simulink library "tqd"  (R2021b)
settings: Solver=VariableStepAuto  StartTime=0.0  StopTime=10.0  RelTol=1e-3
undefined symbols (not defined in the file or in its folder): ATQD_APSDecReq_X_kph, ATQD_APSDecReq_Y_mps2, ATQD_APSDecReqCMD_X_kph, ATQD_APSDecReqTs_X_pct, ATQD_APSDecTimeGain_X_Deg, ATQD_APSDecTimeGain_Y_s, ATQD_APSReqLowSpd_X_Deg, ATQD_AutoHoldReleaseBPS_X_Deg, ATQD_AWDLoadTrqnsGain_X_kg, ATQD_AWDLoadTrqnsGain_Y_pct, ATQD_BOSEnBPSPosn_X_kph, ATQD_BOSMap_X_rpm, ATQD_BOSMap_Y_pct, ATQD_CreepBaseTqD_X_kph, ATQD_CreepBaseTqD_Y_Deg, ATQD_CreepBaseTqR_X_kph, ATQD_CreepBaseTqR_Y_Deg, ATQD_CreepBPSDisPosn_X_Deg, ATQD_CreepBPSDisPosnR_X_Deg, ATQD_CreepBPSEnPosn_X_Deg, ATQD_CreepBPSEnPosnR_X_Deg, ATQD_CreepDeltaTq_X_kph, ATQD_CreepIterm_X_kph, ATQD_CreepIterm_Y_kph, ATQD_CreepItermMaxLimit_X_pct, ATQD_CreepPreloadTime_X_kph, ATQD_CreepPreloadTq_X_kph, ATQD_CreepPreloadTq_Y_s, ATQD_CreepProtTq_X_Deg, ATQD_CreepPterm_X_kph, ATQD_ECOTqMapD_X_rpm, ATQD_ECOTqMapD_Y_pct, ATQD_EOPDTqMapDCon_X_rpm, ATQD_EOPDTqMapDCon_Y_Deg, ATQD_EstInitVehWeight_X_c, ATQD_LHMRollGenMapD_X_rpm, ATQD_LHMRollGenMapD_Y_rpm, ATQD_LHMTqMapD_X_rpm, ATQD_LHMTqMapD_Y_pct, ATQD_NL1TqMapD_X_rpm, ATQD_NL1TqMapD_Y_pct, ATQD_NOPDTqMapDCon_X_rpm, ATQD_NOPDTqMapDCon_Y_Deg, ATQD_NRMRrEDUSpRat_X_rpm, ATQD_NRMRrEDUSpRat_Y_Nm, ATQD_OPDHoldDownRelDelay_X_Deg, ATQD_OPDHoldEnSpd_X_Deg, ATQD_OPDHoldRelDetTime_X_Deg, ATQD_OPDHoldReleaseTq_X_Deg, ATQD_OrigPedTqLowLim_X_Deg, ATQD_OrigPedTqLowLim_Y_pct, ATQD_PedalMapClimbUpLim_X_rpm, ATQD_PedalMapClimbUpLim_Y_Deg, ATQD_PreLoadTq_X_s, ATQD_RollGenMapEL1_X_rpm, ATQD_RollGenMapEL1_Y_rpm, ATQD_SL1TqMapD_X_rpm, ATQD_SL1TqMapD_Y_pct, ATQD_SlideRegenTqGain_X_Gps, ATQD_SlideRegenTqGain_Y_pct ... (+444)
libraries: hcu_lib x70, simulink x61, tqr x1
(part 12 of 14)

== system tqd/TQD/TorqueDemand/TorqueModule/DriverWhlTqDem/Creep/If Action Subsystem1 ==
  VTQD_ActBPSPosnInRange_flg : Inport
  VTQD_CreepErrSpd_kph : Inport  Port=2
  VTQD_CreepPterm_c : Inport  Port=3
  VTQD_CreepIterm_c : Inport  Port=4
  VTQD_CreepDeltaTq_Nm : Inport  Port=5
  VTQD_ActBPSPosn_pct : Inport  Port=6
  task_time_s : Inport  Port=7
  VTQD_CreepDisable_flg : Inport  Port=8
  VTQD_CreepEnable_flg : Inport  Port=9
  VTQD_OPDOn2Off : Inport  Port=10
  Add : Sum
  Add1 : Sum  Inputs=+++
  Constant : Constant  Value=ZERO_FLOAT
  Constant1 : Constant  Value=KTQD_CreepItermMinLimit_Nm
  Constant4 : Constant  Value=ZERO_FLOAT
  Constant5 : Constant  Value=ONE_FLOAT
  Data Type Conversion : DataTypeConversion
  Goto1 : Goto  Commented=on  GotoTag=VTQD_CreepErrSpd_kph
  Goto10 : Goto  Commented=on  GotoTag=VTQD_CreepTotalOfstTq_Nm
  Goto6 : Goto  Commented=on  GotoTag=task_time_s
  Goto7 : Goto  Commented=on  GotoTag=VTQD_CreepPtermTq_Nm
  Goto8 : Goto  Commented=on  GotoTag=VTQD_CreepItermTq_Nm
  Goto9 : Goto  Commented=on  GotoTag=VTQD_CreepOffsetTq_Nm
  Ground{1..6} (6 alike) : Ground  Commented=on
  MTQD_CreepItermMaxLimit_Y_Nm : Lookup_n-D  NumberOfTableDimensions=1  BreakpointsForDimension1=ATQD_CreepItermMaxLimit_X_pct  Table=MTQD_CreepItermMaxLimit_Y_Nm  ExtrapMethod=Clip  InternalRulePriority=Speed  RndMeth=Simplest  InputSameDT=on
  NOT : Logic  Operator=NOT  AllPortsSameDT=off  OutDataTypeStr=boolean
  OR : Logic  Operator=OR  Inputs=4  AllPortsSameDT=off  OutDataTypeStr=boolean
  Product : Product
  Product2 : Product
  Saturation Dynamic : simulink/Discontinuities/Saturation Dynamic  OutMin=[]  OutMax=[]  OutDataTypeStr=Inherit: Same as second input  OutDataType=fixdt(1, 16)  OutScaling=2^-10  DoSatur=off
  Switch1 : Switch  Criteria=u2 ~= 0
  Switch4 : Switch  Criteria=u2 ~= 0
  Terminator1 : Terminator
  Terminator2 : Terminator
  Unit Delay : UnitDelay  SampleTime=-1  HasFrameUpgradeWarning=on
  VTQD_CreepTotalOfstTq_Nm : Outport
  wires:
  Add1/1 -> VTQD_CreepTotalOfstTq_Nm/1  "VTQD_CreepTotalOfstTq_Nm"
  VTQD_CreepDeltaTq_Nm/1 -> [VTQD_CreepDeltaTq_Nm]
  VTQD_CreepIterm_c/1 -> [VTQD_CreepIterm_c]
  VTQD_CreepPterm_c/1 -> [VTQD_CreepPterm_c]
  VTQD_ActBPSPosnInRange_flg/1 -> [VTQD_ActBPSPosnInRange_flg]
  task_time_s/1 -> Terminator1/1
  VTQD_ActBPSPosn_pct/1 -> [VTQD_ActBPSPosn_pct]
  Ground1/1 -> Goto6/1
  Ground2/1 -> Goto7/1
  Ground3/1 -> Goto8/1
  Ground4/1 -> Goto9/1
  Ground5/1 -> Goto10/1
  VTQD_CreepErrSpd_kph/1 -> Terminator2/1
  Ground6/1 -> Goto1/1
  VTQD_CreepDisable_flg/1 -> [VTQD_CreepDisable_flg]
  OR/1 -> [VTQD_CreepPICtrlReset_flg]  "VTQD_CreepPICtrlReset_flg"
  VTQD_CreepEnable_flg/1 -> [VTQD_CreepEnable_flg]
  VTQD_OPDOn2Off/1 -> [VTQD_OPDOn2Off_flg]
  [VTQD_OPDOn2Off_flg] -> OR/2
  [VTQD_CreepDisable_flg] -> OR/3
  [VTQD_ActBPSPosnInRange_flg] -> OR/1
  [VTQD_CreepEnable_flg] -> NOT/1
  NOT/1 -> OR/4
  Data Type Conversion/1 -> Add1/3  "VTQD_CreepOffsetTq_Nm"
  Constant1/1 -> Saturation Dynamic/3
  [VTQD_ActBPSPosn_pct] -> MTQD_CreepItermMaxLimit_Y_Nm/1
  [VTQD_CreepPICtrlReset_flg] -> Switch4/2
  MTQD_CreepItermMaxLimit_Y_Nm/1 -> Saturation Dynamic/1  "VTQD_CreepItermMaxLimit_Nm"
  Constant/1 -> Switch1/1
  Product/1 -> Switch1/3
  [VTQD_CreepPterm_c] -> Product/1
  Constant5/1 -> Product/2, Product2/1
  [VTQD_CreepPICtrlReset_flg] -> Switch1/2
  Add/1 -> Switch4/3
  Switch1/1 -> Add1/1  "VTQD_CreepPtermTq_Nm"
  Saturation Dynamic/1 -> Add1/2  "VTQD_CreepItermTq_Nm"
  Product2/1 -> Add/1
  Switch4/1 -> Unit Delay/1, Saturation Dynamic/2
  Unit Delay/1 -> Add/2
  Constant4/1 -> Switch4/1
  [VTQD_CreepIterm_c] -> Product2/2
  [VTQD_CreepDeltaTq_Nm] -> Data Type Conversion/1

== system tqd/TQD/TorqueDemand/TorqueModule/DriverWhlTqDem/Creep/Switch Case Action Subsystem ==
  In1 : Inport
  Action Port : ActionPort
  Out1 : Outport
  wires:
  In1/1 -> Out1/1

== system tqd/TQD/TorqueDemand/TorqueModule/DriverWhlTqDem/PedalMapWhlTq/LHM ==
  VTQD_ActAPSPosn_pct : Inport
  VTQD_TqTargetShaftSpd_rpm : Inport  Port=2
  VTQD_RollRegenEnable_flg : Inport  Port=3
  VTQD_RollingShaftSpd_rpm : Inport  Port=4
  VTQD_GearActualPosn_enum : Inport  Port=5
  Action Port : ActionPort
  Constant : Constant  Value=ZERO_FLOAT
  Constant1 : Constant  Value=ENUM_GEARACTUALPOSN_D
  Constant11 : Constant  Commented=on  Value=ENUM_GEARACTUALPOSN_D
  Constant12 : Constant  Commented=on  Value=ENUM_GEARACTUALPOSN_R
  Constant2 : Constant  Value=ENUM_GEARACTUALPOSN_R
  Equal1 : RelationalOperator  Operator===  OutDataTypeStr=boolean  RndMeth=Simplest
  Equal2 : RelationalOperator  Operator===  OutDataTypeStr=boolean  RndMeth=Simplest
  Equal7 : RelationalOperator  Commented=on  Operator===  OutDataTypeStr=boolean  RndMeth=Simplest
  Equal8 : RelationalOperator  Commented=on  Operator===  OutDataTypeStr=boolean  RndMeth=Simplest
  From22 : From  Commented=on  GotoTag=VTQD_GearActualPosn_enum
  From23 : From  Commented=on  GotoTag=VTQD_GearActualPosn_enum
  From24 : From  Commented=on  GotoTag=VTQD_ActAPSPosn_pct
  From25 : From  Commented=on  GotoTag=VTQD_TqTargetShaftSpd_rpm
  From39 : From  Commented=on  GotoTag=VTQD_ActAPSPosn_pct
  From40 : From  Commented=on  GotoTag=VTQD_TqTargetShaftSpd_rpm
  From8 : From  Commented=on  GotoTag=VTQD_RollRegenEnable_flg
  From9 : From  Commented=on  GotoTag=VTQD_RollingShaftSpd_rpm
  GearShiftCheck : If  Commented=on  NumInputs=2  IfExpression=u1~= 0  ElseIfExpressions=u2~= 0
  MTQD_LHMRollGenMapD_Z_Nm : Lookup_n-D  BreakpointsForDimension1=ATQD_RollGenMapEL1_Y_rpm  BreakpointsForDimension2=ATQD_RollGenMapEL1_X_rpm  Table=MTQD_LHMRollGenMapD_Z_Nm  ExtrapMethod=Clip  InternalRulePriority=Speed  RndMeth=Simplest  InputSameDT=on
      settings: InputPortMap=u0,u1
  MTQD_LHMTqMapD_Z_Nm : Lookup_n-D  BreakpointsForDimension1=ATQD_NL1TqMapD_Y_pct  BreakpointsForDimension2=ATQD_NL1TqMapD_X_rpm  Table=MTQD_LHMTqMapD_Z_Nm  ExtrapMethod=Clip  InternalRulePriority=Speed  RndMeth=Simplest  InputSameDT=on
      settings: InputPortMap=u0,u1
  MTQD_LHMTqMapR_Z_Nm : Lookup_n-D  BreakpointsForDimension1=ATQD_NL1TqMapD_Y_pct  BreakpointsForDimension2=ATQD_NL1TqMapD_X_rpm  Table=MTQD_LHMTqMapR_Z_Nm  ExtrapMethod=Clip  InternalRulePriority=Speed  RndMeth=Simplest  InputSameDT=on
      settings: InputPortMap=u0,u1
  Merge1 : Merge  Commented=on  Inputs=3
  ShiftD : Subsystem  Commented=on  TreatAsAtomicUnit=on
  ShiftPorN : Subsystem  Commented=on  TreatAsAtomicUnit=on
  ShiftR : Subsystem  Commented=on  TreatAsAtomicUnit=on
  Switch1 : Switch  Criteria=u2 ~= 0
  Switch2 : Switch  Criteria=u2 ~= 0
  Terminator : Terminator
  Terminator1 : Terminator
  VTQD_PedalMapWhlTqLHM_Nm : Outport
  wires:
  Switch1/1 -> VTQD_PedalMapWhlTqLHM_Nm/1
  Constant/1 -> Switch2/3
  [VTQD_LHMTqMapR_Nm] -> Switch2/1
  Equal2/1 -> Switch2/2
  Constant2/1 -> Equal2/2
  [VTQD_GearActualPosn_enum] -> Equal2/1
  Switch2/1 -> Switch1/3
  [VTQD_LHMTqMapD_Nm] -> Switch1/1
  Constant1/1 -> Equal1/2
  Equal1/1 -> Switch1/2
  [VTQD_GearActualPosn_enum] -> Equal1/1
  [VTQD_TqTargetShaftSpd_rpm] -> MTQD_LHMTqMapR_Z_Nm/2
  [VTQD_ActAPSPosn_pct] -> MTQD_LHMTqMapR_Z_Nm/1
  MTQD_LHMTqMapR_Z_Nm/1 -> [VTQD_LHMTqMapR_Nm]
  MTQD_LHMRollGenMapD_Z_Nm/1 -> Terminator1/1
  [VTQD_TqTargetShaftSpd_rpm] -> MTQD_LHMRollGenMapD_Z_Nm/2
  MTQD_LHMTqMapD_Z_Nm/1 -> [VTQD_LHMTqMapD_Nm]
  [VTQD_TqTargetShaftSpd_rpm] -> MTQD_LHMTqMapD_Z_Nm/2
  [VTQD_ActAPSPosn_pct] -> MTQD_LHMTqMapD_Z_Nm/1
  [VTQD_RollingShaftSpd_rpm] -> MTQD_LHMRollGenMapD_Z_Nm/1
  VTQD_GearActualPosn_enum/1 -> [VTQD_GearActualPosn_enum]
  VTQD_RollingShaftSpd_rpm/1 -> [VTQD_RollingShaftSpd_rpm]
  VTQD_RollRegenEnable_flg/1 -> Terminator/1
  VTQD_TqTargetShaftSpd_rpm/1 -> [VTQD_TqTargetShaftSpd_rpm]
  VTQD_ActAPSPosn_pct/1 -> [VTQD_ActAPSPosn_pct]
  From25/1 -> ShiftR/2(VTQD_TqTargetShaftSpd_rpm)
  Constant12/1 -> Equal8/2
  From9/1 -> ShiftD/4(VTQD_RollingShaftSpd_rpm)
  GearShiftCheck/1 -> ShiftD/Action
  GearShiftCheck/3 -> ShiftPorN/Action
  Equal7/1 -> GearShiftCheck/1
  Constant11/1 -> Equal7/2
  ShiftD/1(VTQD_PedalMapWhlTqLHMD_Nm) -> Merge1/1
  From23/1 -> Equal8/1
  From39/1 -> ShiftD/1(VTQD_ActAPSPosn_pct)
  From22/1 -> Equal7/1
  GearShiftCheck/2 -> ShiftR/Action
  From8/1 -> ShiftD/3(VTQD_RollRegenEnable_flg)
  From40/1 -> ShiftD/2(VTQD_TqTargetShaftSpd_rpm)
  ShiftPorN/1(VTQD_PedalMapWhlTqPorN_Nm) -> Merge1/3
  From24/1 -> ShiftR/1(VTQD_ActAPSPosn_pct)
  Equal8/1 -> GearShiftCheck/2
  ShiftR/1(VTQD_PedalMapWhlTqLHMR_Nm) -> Merge1/2

== system tqd/TQD/TorqueDemand/TorqueModule/DriverWhlTqDem/PedalMapWhlTq/NoLHM ==
  VTQD_ActAPSPosn_pct : Inport
  VTQD_TqTargetShaftSpd_rpm : Inport  Port=2
  VTQD_RegenMode_enum : Inport  Port=3
  VTQD_RollRegenEnable_flg : Inport  Port=4
  VTQD_RollingShaftSpd_rpm : Inport  Port=5
  VTQD_GearActualPosn_enum : Inport  Port=6
  VTQD_EVDriveMode_enum : Inport  Port=7
  VVMC_EstSlope_Deg : Inport  Port=8
  VTQD_APSReqTimer_s : Inport  Port=9
  VTQD_LowIdleAccPedal_flg : Inport  Port=10
  VTQD_OPDHoldEnRel_flg : Inport  Port=11
  VTQD_OPDHoldActRelTq_Nm : Inport  Port=12
  VTQD_VehActSpd_kph : Inport  Port=13
  Action Port : ActionPort
  Constant11 : Constant  Value=ENUM_GEARACTUALPOSN_D
  Constant12 : Constant  Value=ENUM_GEARACTUALPOSN_R
  Equal7 : RelationalOperator  Operator===  OutDataTypeStr=boolean  RndMeth=Simplest
  Equal8 : RelationalOperator  Operator===  OutDataTypeStr=boolean  RndMeth=Simplest
  GearShiftCheck : If  NumInputs=2  IfExpression=u1~= 0  ElseIfExpressions=u2~= 0
  Merge1 : Merge  Inputs=3
  ShiftD : Subsystem  TreatAsAtomicUnit=on
  ShiftPorN : Subsystem  TreatAsAtomicUnit=on
  ShiftR : Subsystem  TreatAsAtomicUnit=on
  VTQD_PedalMapWhlTqNoLHM_Nm : Outport
  wires:
  [VTQD_RollingShaftSpd_rpm] -> ShiftD/6(VTQD_RollingShaftSpd_rpm)
  [VTQD_RollRegenEnable_flg] -> ShiftD/5(VTQD_RollRegenEnable_flg)
  ShiftR/1(VTQD_PedalMapWhlTqR_Nm) -> Merge1/2
  VTQD_EVDriveMode_enum/1 -> [VTQD_EVDriveMode_enum]
  VTQD_GearActualPosn_enum/1 -> [VTQD_GearActualPosn_enum]
  [VTQD_TqTargetShaftSpd_rpm] -> ShiftD/3(VTQD_TqTargetShaftSpd_rpm)
  Equal7/1 -> GearShiftCheck/1
  GearShiftCheck/3 -> ShiftPorN/Action
  Equal8/1 -> GearShiftCheck/2
  [VTQD_ActAPSPosn_pct] -> ShiftR/1(VTQD_ActAPSPosn_pct)
  ShiftPorN/1(VTQD_PedalMapWhlTqPorN_Nm) -> Merge1/3
  [VTQD_EVDriveMode_enum] -> ShiftD/1(VTQD_EVDriveMode_enum)
  [VTQD_TqTargetShaftSpd_rpm] -> ShiftR/2(VTQD_TqTargetShaftSpd_rpm)
  GearShiftCheck/1 -> ShiftD/Action
  Merge1/1 -> VTQD_PedalMapWhlTqNoLHM_Nm/1  "VTQD_PedalMapWhlTqNoLHM_Nm"
  Constant12/1 -> Equal8/2
  Constant11/1 -> Equal7/2
  GearShiftCheck/2 -> ShiftR/Action
  [VTQD_GearActualPosn_enum] -> Equal7/1
  [VTQD_ActAPSPosn_pct] -> ShiftD/2(VTQD_ActAPSPosn_pct)
  [VTQD_GearActualPosn_enum] -> Equal8/1
  ShiftD/1(VTQD_PedalMapWhlTqD_Nm) -> Merge1/1
  VTQD_RollingShaftSpd_rpm/1 -> [VTQD_RollingShaftSpd_rpm]
  VTQD_RollRegenEnable_flg/1 -> [VTQD_RollRegenEnable_flg]
  VTQD_RegenMode_enum/1 -> [VTQD_RegenMode_enum]
  VTQD_ActAPSPosn_pct/1 -> [VTQD_ActAPSPosn_pct]
  VTQD_TqTargetShaftSpd_rpm/1 -> [VTQD_TqTargetShaftSpd_rpm]
  [VVMC_EstSlope_Deg] -> ShiftD/7(VVMC_EstSlope_Deg)
  [VTQD_APSReqTimer_s] -> ShiftD/8(VTQD_APSReqTimer_s)
  VVMC_EstSlope_Deg/1 -> [VVMC_EstSlope_Deg]
  VTQD_APSReqTimer_s/1 -> [VTQD_APSReqTimer_s]
  [VTQD_RegenMode_enum] -> ShiftD/4(VTQD_RegenMode_enum)
  [VTQD_LowIdleAccPedal_flg] -> ShiftD/9(VTQD_LowIdleAccPedal_flg)
  VTQD_LowIdleAccPedal_flg/1 -> [VTQD_LowIdleAccPedal_flg]
  VTQD_OPDHoldEnRel_flg/1 -> [VTQD_OPDHoldEnRel_flg]
  [VTQD_OPDHoldEnRel_flg] -> ShiftD/10(VTQD_OPDHoldEnRel_flg)
  VTQD_OPDHoldActRelTq_Nm/1 -> [VTQD_OPDHoldActRelTq_Nm]
  VTQD_VehActSpd_kph/1 -> [VTQD_VehActSpd_kph]
  [VTQD_OPDHoldActRelTq_Nm] -> ShiftD/11(VTQD_OPDHoldActRelTq_Nm)
  [VTQD_VehActSpd_kph] -> ShiftD/12(VTQD_VehActSpd_kph)

== system tqd/TQD/TorqueDemand/TorqueModule/DriverWhlTqDem/PedalMapWhlTq/Triggered Subsystem ==
  in1 : Inport
  In2 : Inport  Port=2
  Trigger : TriggerPort  VariantControl=(inherit)
  Out1 : Outport
  Out2 : Outport  Port=2
  wires:
  in1/1 -> Out1/1
  In2/1 -> Out2/1

== system tqd/TQD/TorqueDemand/TorqueModule/DriverWhlTqDem/PedalMapWhlTq/LHM/ShiftD ==
  VTQD_ActAPSPosn_pct : Inport
  VTQD_TqTargetShaftSpd_rpm : Inport  Port=2
  VTQD_RollRegenEnable_flg : Inport  Port=3
  VTQD_RollingShaftSpd_rpm : Inport  Port=4
  Action Port : ActionPort
  MTQD_LHMRollGenMapD_Z_Nm : Lookup_n-D  BreakpointsForDimension1=ATQD_LHMRollGenMapD_Y_rpm  BreakpointsForDimension2=ATQD_LHMRollGenMapD_X_rpm  Table=MTQD_LHMRollGenMapD_Z_Nm  InternalRulePriority=Speed  RndMeth=Simplest  InputSameDT=on
      settings: InputPortMap=u0,u1
  MTQD_LHMTqMapD_Z_Nm : Lookup_n-D  BreakpointsForDimension1=ATQD_LHMTqMapD_Y_pct  BreakpointsForDimension2=ATQD_LHMTqMapD_X_rpm  Table=MTQD_LHMTqMapD_Z_Nm  InternalRulePriority=Speed  RndMeth=Simplest  InputSameDT=on
      settings: InputPortMap=u0,u1
  Switch : Switch  Criteria=u2 ~= 0
  VTQD_PedalMapWhlTqLHMD_Nm : Outport
  wires:
  Switch/1 -> VTQD_PedalMapWhlTqLHMD_Nm/1
  [MTQD_LHMTqMapD_Z_Nm] -> Switch/3
  [MTQD_LHMRollGenMapD_Z_Nm] -> Switch/1
  [VTQD_RollRegenEnable_flg] -> Switch/2
  MTQD_LHMRollGenMapD_Z_Nm/1 -> [MTQD_LHMRollGenMapD_Z_Nm]
  [VTQD_TqTargetShaftSpd_rpm] -> MTQD_LHMRollGenMapD_Z_Nm/2
  [VTQD_RollingShaftSpd_rpm] -> MTQD_LHMRollGenMapD_Z_Nm/1
  [VTQD_TqTargetShaftSpd_rpm] -> MTQD_LHMTqMapD_Z_Nm/2
  [VTQD_ActAPSPosn_pct] -> MTQD_LHMTqMapD_Z_Nm/1
  MTQD_LHMTqMapD_Z_Nm/1 -> [MTQD_LHMTqMapD_Z_Nm]
  VTQD_RollingShaftSpd_rpm/1 -> [VTQD_RollingShaftSpd_rpm]
  VTQD_RollRegenEnable_flg/1 -> [VTQD_RollRegenEnable_flg]
  VTQD_TqTargetShaftSpd_rpm/1 -> [VTQD_TqTargetShaftSpd_rpm]
  VTQD_ActAPSPosn_pct/1 -> [VTQD_ActAPSPosn_pct]

== system tqd/TQD/TorqueDemand/TorqueModule/DriverWhlTqDem/PedalMapWhlTq/LHM/ShiftPorN ==
  Action Port : ActionPort
  Constant : Constant  Value=ZERO_FLOAT
  VTQD_PedalMapWhlTqPorN_Nm : Outport
  wires:
  Constant/1 -> VTQD_PedalMapWhlTqPorN_Nm/1

== system tqd/TQD/TorqueDemand/TorqueModule/DriverWhlTqDem/PedalMapWhlTq/LHM/ShiftR ==
  VTQD_ActAPSPosn_pct : Inport
  VTQD_TqTargetShaftSpd_rpm : Inport  Port=2
  Action Port : ActionPort
  MTQD_LHMTqMapR_Z_Nm : Lookup_n-D  BreakpointsForDimension1=ATQD_LHMTqMapD_Y_pct  BreakpointsForDimension2=ATQD_LHMTqMapD_X_rpm  Table=MTQD_LHMTqMapR_Z_Nm  InternalRulePriority=Speed  RndMeth=Simplest  InputSameDT=on
      settings: InputPortMap=u0,u1
  VTQD_PedalMapWhlTqLHMR_Nm : Outport
  wires:
  [MTQD_LHMTqMapR_Z_Nm] -> VTQD_PedalMapWhlTqLHMR_Nm/1
  MTQD_LHMTqMapR_Z_Nm/1 -> [MTQD_LHMTqMapR_Z_Nm]
  [VTQD_ActAPSPosn_pct] -> MTQD_LHMTqMapR_Z_Nm/1
  [VTQD_TqTargetShaftSpd_rpm] -> MTQD_LHMTqMapR_Z_Nm/2
  VTQD_ActAPSPosn_pct/1 -> [VTQD_ActAPSPosn_pct]
  VTQD_TqTargetShaftSpd_rpm/1 -> [VTQD_TqTargetShaftSpd_rpm]

== system tqd/TQD/TorqueDemand/TorqueModule/DriverWhlTqDem/PedalMapWhlTq/NoLHM/ShiftD ==
  VTQD_EVDriveMode_enum : Inport
  VTQD_ActAPSPosn_pct : Inport  Port=2
  VTQD_TqTargetShaftSpd_rpm : Inport  Port=3
  VTQD_RegenMode_enum : Inport  Port=4
  VTQD_RollRegenEnable_flg : Inport  Port=5
  VTQD_RollingShaftSpd_rpm : Inport  Port=6
  VVMC_EstSlope_Deg : Inport  Port=7
  VTQD_APSReqTimer_s : Inport  Port=8
  VTQD_LowIdleAccPedal_flg : Inport  Port=9
  VTQD_OPDHoldEnRel_flg : Inport  Port=10
  VTQD_OPDHoldActRelTq_Nm : Inport  Port=11
  VTQD_VehActSpd_kph : Inport  Port=12
  Action Port : ActionPort
  Constant5 : Constant  Value=ENUM_DRIVEMODE_NRM
  Constant6 : Constant  Value=ENUM_DRIVEMODE_ECO
  Constant7 : Constant  Value=ENUM_DRIVEMODE_SPORT
  Equal1 : RelationalOperator  Operator===  OutDataTypeStr=boolean  RndMeth=Simplest
  Equal2 : RelationalOperator  Operator===  OutDataTypeStr=boolean  RndMeth=Simplest
  Equal3 : RelationalOperator  Operator===  OutDataTypeStr=boolean  RndMeth=Simplest
  If : If  NumInputs=3  IfExpression=u1 ~= 0  ElseIfExpressions=u2 ~= 0
  LUT_D_ECO : Subsystem  TreatAsAtomicUnit=on
  LUT_D_Normal : Subsystem  TreatAsAtomicUnit=on
  LUT_D_Sport : Subsystem  TreatAsAtomicUnit=on
  Merge : Merge  Inputs=3
  VTQD_PedalMapWhlTqD_Nm : Outport
  wires:
  [VTQD_RollingShaftSpd_rpm] -> LUT_D_ECO/5(VTQD_RollingShaftSpd_rpm)
  [VTQD_RollRegenEnable_flg] -> LUT_D_ECO/4(VTQD_RollRegenEnable_flg)
  VTQD_RollingShaftSpd_rpm/1 -> [VTQD_RollingShaftSpd_rpm]
  VTQD_RollRegenEnable_flg/1 -> [VTQD_RollRegenEnable_flg]
  [VTQD_TqTargetShaftSpd_rpm] -> LUT_D_Sport/1(VTQD_TqTargetShaftSpd_rpm)
  [VTQD_ActAPSPosn_pct] -> LUT_D_Sport/2(VTQD_ActAPSPosn_pct)
  [VTQD_RegenMode_enum] -> LUT_D_Sport/3(VTQD_RegenMode_enum)
  [VTQD_RegenMode_enum] -> LUT_D_ECO/3(VTQD_RegenMode_enum)
  [VTQD_ActAPSPosn_pct] -> LUT_D_ECO/2(VTQD_ActAPSPosn_pct)
  [VTQD_TqTargetShaftSpd_rpm] -> LUT_D_ECO/1(VTQD_TqTargetShaftSpd_rpm)
  LUT_D_Normal/1(VTQD_WhlTqNRMD_Nm) -> Merge/1
  If/3 -> LUT_D_Sport/Action
  If/2 -> LUT_D_ECO/Action
  If/1 -> LUT_D_Normal/Action
  LUT_D_ECO/1(VTQD_WhlTqECOD_Nm) -> Merge/2
  LUT_D_Sport/1(VTQD_WhlTqSPORTD_Nm) -> Merge/3
  Equal3/1 -> If/3
  Equal2/1 -> If/2
  Equal1/1 -> If/1
  [VTQD_ActAPSPosn_pct] -> LUT_D_Normal/2(VTQD_ActAPSPosn_pct)
  [VTQD_TqTargetShaftSpd_rpm] -> LUT_D_Normal/1(VTQD_TqTargetShaftSpd_rpm)
  [VTQD_RegenMode_enum] -> LUT_D_Normal/3(VTQD_RegenMode_enum)
  VTQD_RegenMode_enum/1 -> [VTQD_RegenMode_enum]
  VTQD_TqTargetShaftSpd_rpm/1 -> [VTQD_TqTargetShaftSpd_rpm]
  VTQD_ActAPSPosn_pct/1 -> [VTQD_ActAPSPosn_pct]
  VTQD_EVDriveMode_enum/1 -> [VTQD_EVDriveMode_enum]
  Merge/1 -> VTQD_PedalMapWhlTqD_Nm/1
  Constant7/1 -> Equal3/2
  Constant5/1 -> Equal1/2
  [VTQD_EVDriveMode_enum] -> Equal3/1
  Constant6/1 -> Equal2/2
  [VTQD_EVDriveMode_enum] -> Equal2/1
  [VTQD_EVDriveMode_enum] -> Equal1/1
  [VVMC_EstSlope_Deg] -> LUT_D_Normal/4(VVMC_EstSlope_Deg)
  [VTQD_APSReqTimer_s] -> LUT_D_Normal/5(VTQD_APSReqTimer_s)
  VVMC_EstSlope_Deg/1 -> [VVMC_EstSlope_Deg]
  VTQD_APSReqTimer_s/1 -> [VTQD_APSReqTimer_s]
  [VVMC_EstSlope_Deg] -> LUT_D_ECO/6(VVMC_EstSlope_Deg)
  [VTQD_APSReqTimer_s] -> LUT_D_ECO/7(VTQD_APSReqTimer_s)
  [VVMC_EstSlope_Deg] -> LUT_D_Sport/4(VVMC_EstSlope_Deg)
  [VTQD_APSReqTimer_s] -> LUT_D_Sport/5(VTQD_APSReqTimer_s)
  [VTQD_LowIdleAccPedal_flg] -> LUT_D_Normal/6(VTQD_LowIdleAccPedal_flg)
  VTQD_LowIdleAccPedal_flg/1 -> [VTQD_LowIdleAccPedal_flg]
  [VTQD_LowIdleAccPedal_flg] -> LUT_D_ECO/8(VTQD_LowIdleAccPedal_flg)
  [VTQD_LowIdleAccPedal_flg] -> LUT_D_Sport/6(VTQD_LowIdleAccPedal_flg)
  VTQD_OPDHoldEnRel_flg/1 -> [VTQD_OPDHoldEnRel_flg]
  [VTQD_OPDHoldEnRel_flg] -> LUT_D_Normal/7(VTQD_OPDHoldEnRel_flg)
  VTQD_OPDHoldActRelTq_Nm/1 -> [VTQD_OPDHoldActRelTq_Nm]
  VTQD_VehActSpd_kph/1 -> [VTQD_VehActSpd_kph]
  [VTQD_VehActSpd_kph] -> LUT_D_Normal/9(VTQD_VehActSpd_kph)
  [VTQD_OPDHoldActRelTq_Nm] -> LUT_D_Normal/8(VTQD_OPDHoldActRelTq_Nm)
  [VTQD_OPDHoldEnRel_flg] -> LUT_D_ECO/9(VTQD_OPDHoldEnRel_flg)
  [VTQD_OPDHoldActRelTq_Nm] -> LUT_D_ECO/10(VTQD_OPDHoldActRelTq_Nm)
  [VTQD_VehActSpd_kph] -> LUT_D_ECO/11(VTQD_VehActSpd_kph)
  [VTQD_VehActSpd_kph] -> LUT_D_Sport/9(VTQD_VehActSpd_kph)
  [VTQD_OPDHoldActRelTq_Nm] -> LUT_D_Sport/8(VTQD_OPDHoldActRelTq_Nm)
  [VTQD_OPDHoldEnRel_flg] -> LUT_D_Sport/7(VTQD_OPDHoldEnRel_flg)

== system tqd/TQD/TorqueDemand/TorqueModule/DriverWhlTqDem/PedalMapWhlTq/NoLHM/ShiftPorN ==
  Action Port : ActionPort
  Constant : Constant  Value=ZERO_FLOAT
  VTQD_PedalMapWhlTqPorN_Nm : Outport
  wires:
  Constant/1 -> VTQD_PedalMapWhlTqPorN_Nm/1

== system tqd/TQD/TorqueDemand/TorqueModule/DriverWhlTqDem/PedalMapWhlTq/NoLHM/ShiftR ==
  VTQD_ActAPSPosn_pct : Inport
  VTQD_TqTargetShaftSpd_rpm : Inport  Port=2
  Action Port : ActionPort
  MTQD_NRMTqMapR_Z_Nm : Lookup_n-D  BreakpointsForDimension1=ATQD_NL1TqMapD_Y_pct  BreakpointsForDimension2=ATQD_NL1TqMapD_X_rpm  Table=MTQD_NRMTqMapR_Z_Nm  ExtrapMethod=Clip  InternalRulePriority=Speed  RndMeth=Simplest  InputSameDT=on
      settings: InputPortMap=u0,u1
  VTQD_PedalMapWhlTqR_Nm : Outport
  wires:
  [VTQD_NRMTqMapR_Nm] -> VTQD_PedalMapWhlTqR_Nm/1
  MTQD_NRMTqMapR_Z_Nm/1 -> [VTQD_NRMTqMapR_Nm]
  [VTQD_ActAPSPosn_pct] -> MTQD_NRMTqMapR_Z_Nm/1
  [VTQD_TqTargetShaftSpd_rpm] -> MTQD_NRMTqMapR_Z_Nm/2
  VTQD_ActAPSPosn_pct/1 -> [VTQD_ActAPSPosn_pct]
  VTQD_TqTargetShaftSpd_rpm/1 -> [VTQD_TqTargetShaftSpd_rpm]

== system tqd/TQD/TorqueDemand/TorqueModule/DriverWhlTqDem/PedalMapWhlTq/NoLHM/ShiftD/LUT_D_ECO ==
  VTQD_TqTargetShaftSpd_rpm : Inport
  VTQD_ActAPSPosn_pct : Inport  Port=2
  VTQD_RegenMode_enum : Inport  Port=3
  VTQD_RollRegenEnable_flg : Inport  Port=4
  VTQD_RollingShaftSpd_rpm : Inport  Port=5
  VVMC_EstSlope_Deg : Inport  Port=6
  VTQD_APSReqTimer_s : Inport  Port=7
  VTQD_LowIdleAccPedal_flg : Inport  Port=8
  VTQD_OPDHoldEnRel_flg : Inport  Port=9
  VTQD_OPDHoldActRelTq_Nm : Inport  Port=10
  VTQD_VehActSpd_kph : Inport  Port=11
  Action Port : ActionPort
  Constant : Constant  Value=ENUM_REGENLEVEL_LV1
  Constant1 : Constant  Value=ENUM_REGENLEVEL_LV2
  Constant2 : Constant  Value=ENUM_REGENLEVEL_LV3
  Constant3 : Constant  Value=ENUM_REGENLEVEL_LV4
  Constant4 : Constant  Value=ENUM_REGENLEVEL_LV5
  Constant5 : Constant  Value=ENUM_REGENLEVEL_OPD
  ECO_Invalid_TqMap1 : Subsystem  TreatAsAtomicUnit=on
  ECO_Lv1_TqMap : Subsystem  TreatAsAtomicUnit=on
  ECO_Lv2_TqMap : Subsystem  TreatAsAtomicUnit=on
  ECO_Lv3_TqMap : Subsystem  TreatAsAtomicUnit=on
  ECO_Lv4_TqMap : Subsystem  TreatAsAtomicUnit=on
  ECO_Lv5_TqMap : Subsystem  TreatAsAtomicUnit=on
  ECO_OnePedal_TqMap : Subsystem  TreatAsAtomicUnit=on
  Equal{1..6} (6 alike) : RelationalOperator  Operator===  OutDataTypeStr=boolean  RndMeth=Simplest
  If : If  NumInputs=6  IfExpression=u1 ~= 0  ElseIfExpressions=u2 ~= 0, u3 ~= 0, u4 ~= 0, u5 ~= 0, u6 ~= 0
  MTQD_ECOTqMapD_Z_Nm : Lookup_n-D  BreakpointsForDimension1=ATQD_ECOTqMapD_Y_pct  BreakpointsForDimension2=ATQD_ECOTqMapD_X_rpm  Table=MTQD_ECOTqMapD_Z_Nm  ExtrapMethod=Clip  InternalRulePriority=Speed  RndMeth=Simplest  InputSameDT=on
      settings: InputPortMap=u0,u1
  MTQD_EL2TqMapD_Z_Nm : Lookup_n-D  BreakpointsForDimension1=ATQD_ECOTqMapD_Y_pct  BreakpointsForDimension2=ATQD_ECOTqMapD_X_rpm  Table=MTQD_EL2TqMapD_Z_Nm  ExtrapMethod=Clip  InternalRulePriority=Speed  RndMeth=Simplest  InputSameDT=on
      settings: InputPortMap=u0,u1
  MTQD_EL3TqMapD_Z_Nm : Lookup_n-D  BreakpointsForDimension1=ATQD_ECOTqMapD_Y_pct  BreakpointsForDimension2=ATQD_ECOTqMapD_X_rpm  Table=MTQD_EL3TqMapD_Z_Nm  ExtrapMethod=Clip  InternalRulePriority=Speed  RndMeth=Simplest  InputSameDT=on
      settings: InputPortMap=u0,u1
  MTQD_EL4TqMapD_Z_Nm : Lookup_n-D  BreakpointsForDimension1=ATQD_ECOTqMapD_Y_pct  BreakpointsForDimension2=ATQD_ECOTqMapD_X_rpm  Table=MTQD_EL4TqMapD_Z_Nm  ExtrapMethod=Clip  InternalRulePriority=Speed  RndMeth=Simplest  InputSameDT=on
      settings: InputPortMap=u0,u1
  MTQD_EL5TqMapD_Z_Nm : Lookup_n-D  BreakpointsForDimension1=ATQD_ECOTqMapD_Y_pct  BreakpointsForDimension2=ATQD_ECOTqMapD_X_rpm  Table=MTQD_EL5TqMapD_Z_Nm  ExtrapMethod=Clip  InternalRulePriority=Speed  RndMeth=Simplest  InputSameDT=on
      settings: InputPortMap=u0,u1
  MTQD_EOPDTqMapDCon_Z_Nm : Lookup_n-D  BreakpointsForDimension1=ATQD_EOPDTqMapDCon_Y_Deg  BreakpointsForDimension2=ATQD_EOPDTqMapDCon_X_rpm  Table=MTQD_EOPDTqMapDCon_Z_Nm  ExtrapMethod=Clip  InternalRulePriority=Speed  RndMeth=Simplest  InputSameDT=on
      settings: InputPortMap=u0,u1
  MTQD_EOPDTqMapD_Z_Nm : Lookup_n-D  BreakpointsForDimension1=ATQD_ECOTqMapD_Y_pct  BreakpointsForDimension2=ATQD_ECOTqMapD_X_rpm  Table=MTQD_EOPDTqMapD_Z_Nm  ExtrapMethod=Clip  InternalRulePriority=Speed  RndMeth=Simplest  InputSameDT=on
      settings: InputPortMap=u0,u1
  MTQD_RollGenMapEL1_Z_Nm : Lookup_n-D  BreakpointsForDimension1=ATQD_RollGenMapEL1_Y_rpm  BreakpointsForDimension2=ATQD_RollGenMapEL1_X_rpm  Table=MTQD_RollGenMapEL1_Z_Nm  ExtrapMethod=Clip  InternalRulePriority=Speed  RndMeth=Simplest  InputSameDT=on
      settings: InputPortMap=u0,u1
  Merge : Merge  Inputs=7
  VTQD_WhlTqECOD_Nm : Outport
  wires:
  [VTQD_ECOTqMapD_Nm] -> ECO_Lv1_TqMap/3(MTQD_ECOTqMapD_Z_Nm)
  [VTQD_RollGenMapEL1_Nm] -> ECO_Lv1_TqMap/2(MTQD_RollGenMapEL1_Z_Nm)
  [VTQD_RollRegenEnable_flg] -> ECO_Lv1_TqMap/1(VTQD_RollRegenEnable_flg)
  [VTQD_TqTargetShaftSpd_rpm] -> MTQD_RollGenMapEL1_Z_Nm/2
  [VTQD_RollingShaftSpd_rpm] -> MTQD_RollGenMapEL1_Z_Nm/1
  MTQD_RollGenMapEL1_Z_Nm/1 -> [VTQD_RollGenMapEL1_Nm]
  VTQD_RollingShaftSpd_rpm/1 -> [VTQD_RollingShaftSpd_rpm]
  VTQD_RollRegenEnable_flg/1 -> [VTQD_RollRegenEnable_flg]
  Equal6/1 -> If/6
  [VTQD_RegenMode_enum] -> Equal6/1
  Constant5/1 -> Equal6/2
  Equal5/1 -> If/5
  [VTQD_RegenMode_enum] -> Equal5/1
  Constant4/1 -> Equal5/2
  Equal4/1 -> If/4
  [VTQD_RegenMode_enum] -> Equal4/1
  Constant3/1 -> Equal4/2
  [VTQD_RegenMode_enum] -> Equal3/1
  Constant2/1 -> Equal3/2
  [VTQD_RegenMode_enum] -> Equal2/1
  Constant1/1 -> Equal2/2
  Constant/1 -> Equal1/2
  [VTQD_RegenMode_enum] -> Equal1/1
  [VTQD_EOPDTqMapD_Nm] -> ECO_OnePedal_TqMap/1(VTQD_EOPDTqMapDIn_Nm)
  If/6 -> ECO_OnePedal_TqMap/Action
  ECO_OnePedal_TqMap/1(VTQD_EOPDTqMapDOut_Nm) -> Merge/6
  [VTQD_EL5TqMapD_Nm] -> ECO_Lv5_TqMap/1(VTQD_EL5TqMapDIn_Nm)
  If/5 -> ECO_Lv5_TqMap/Action
  ECO_Lv5_TqMap/1(VTQD_EL5TqMapDOut_Nm) -> Merge/5
  ECO_Lv4_TqMap/1(VTQD_EL4TqMapDOut_Nm) -> Merge/4
  If/4 -> ECO_Lv4_TqMap/Action
  [VTQD_EL4TqMapD_Nm] -> ECO_Lv4_TqMap/1(VTQD_EL4TqMapDIn_Nm)
  [VTQD_EL3TqMapD_Nm] -> ECO_Lv3_TqMap/1(VTQD_EL3TqMapDIn_Nm)
  If/3 -> ECO_Lv3_TqMap/Action
  ECO_Lv3_TqMap/1(VTQD_EL3TqMapDOut_Nm) -> Merge/3
  [VTQD_EL2TqMapD_Nm] -> ECO_Lv2_TqMap/1(VTQD_EL2TqMapDIn_Nm)
  ECO_Lv2_TqMap/1(VTQD_EL2TqMapDOut_Nm) -> Merge/2
  If/2 -> ECO_Lv2_TqMap/Action
  ECO_Lv1_TqMap/1(VTQD_EL1TqMapDOut_Nm) -> Merge/1
  Equal1/1 -> If/1
  Equal2/1 -> If/2
  If/1 -> ECO_Lv1_TqMap/Action
  Merge/1 -> VTQD_WhlTqECOD_Nm/1
  Equal3/1 -> If/3
  [VTQD_TqTargetShaftSpd_rpm] -> MTQD_EOPDTqMapD_Z_Nm/2
  [VTQD_ActAPSPosn_pct] -> MTQD_EOPDTqMapD_Z_Nm/1
  [VTQD_TqTargetShaftSpd_rpm] -> MTQD_EL5TqMapD_Z_Nm/2
  [VTQD_ActAPSPosn_pct] -> MTQD_EL5TqMapD_Z_Nm/1
  [VTQD_TqTargetShaftSpd_rpm] -> MTQD_EL3TqMapD_Z_Nm/2
  [VTQD_ActAPSPosn_pct] -> MTQD_EL3TqMapD_Z_Nm/1
  [VTQD_TqTargetShaftSpd_rpm] -> MTQD_EL2TqMapD_Z_Nm/2
  [VTQD_ActAPSPosn_pct] -> MTQD_EL2TqMapD_Z_Nm/1
  MTQD_EL5TqMapD_Z_Nm/1 -> [VTQD_EL5TqMapD_Nm]
  MTQD_EL4TqMapD_Z_Nm/1 -> [VTQD_EL4TqMapD_Nm]
  [VTQD_TqTargetShaftSpd_rpm] -> MTQD_EL4TqMapD_Z_Nm/2
  [VTQD_ActAPSPosn_pct] -> MTQD_EL4TqMapD_Z_Nm/1
  MTQD_EOPDTqMapD_Z_Nm/1 -> [VTQD_EOPDTqMapD_Nm]
  MTQD_EL3TqMapD_Z_Nm/1 -> [VTQD_EL3TqMapD_Nm]
  MTQD_EL2TqMapD_Z_Nm/1 -> [VTQD_EL2TqMapD_Nm]
  [VTQD_ActAPSPosn_pct] -> MTQD_ECOTqMapD_Z_Nm/1
  [VTQD_TqTargetShaftSpd_rpm] -> MTQD_ECOTqMapD_Z_Nm/2
  VTQD_RegenMode_enum/1 -> [VTQD_RegenMode_enum]
  VTQD_ActAPSPosn_pct/1 -> [VTQD_ActAPSPosn_pct]
  VTQD_TqTargetShaftSpd_rpm/1 -> [VTQD_TqTargetShaftSpd_rpm]
  MTQD_ECOTqMapD_Z_Nm/1 -> [VTQD_ECOTqMapD_Nm]
  ECO_Invalid_TqMap1/1(VTQD_EL1TqMapDOut_Nm) -> Merge/7
  [VTQD_RollRegenEnable_flg] -> ECO_Invalid_TqMap1/1(VTQD_RollRegenEnable_flg)
  [VTQD_RollGenMapEL1_Nm] -> ECO_Invalid_TqMap1/2(MTQD_RollGenMapEL1_Z_Nm)
  [VTQD_ECOTqMapD_Nm] -> ECO_Invalid_TqMap1/3(MTQD_ECOTqMapD_Z_Nm)
  If/7 -> ECO_Invalid_TqMap1/Action
  [VTQD_TqTargetShaftSpd_rpm] -> MTQD_EOPDTqMapDCon_Z_Nm/2
  [VVMC_EstSlope_Deg] -> MTQD_EOPDTqMapDCon_Z_Nm/1
  MTQD_EOPDTqMapDCon_Z_Nm/1 -> [VTQD_EOPDTqMapDCon_Nm]
  VVMC_EstSlope_Deg/1 -> [VVMC_EstSlope_Deg]
  VTQD_APSReqTimer_s/1 -> [VTQD_APSReqTimer_s]
  [VTQD_EOPDTqMapDCon_Nm] -> ECO_OnePedal_TqMap/2(VTQD_EOPDTqMapDCon_Nm)
  [VTQD_APSReqTimer_s] -> ECO_OnePedal_TqMap/3(VTQD_APSReqTimer_s)
  [VTQD_LowIdleAccPedal_flg] -> ECO_OnePedal_TqMap/4(VTQD_LowIdleAccPedal_flg)
  VTQD_LowIdleAccPedal_flg/1 -> [VTQD_LowIdleAccPedal_flg]
  VTQD_OPDHoldActRelTq_Nm/1 -> [VTQD_OPDHoldActRelTq_Nm]
  VTQD_OPDHoldEnRel_flg/1 -> [VTQD_OPDHoldEnRel_flg]
  VTQD_VehActSpd_kph/1 -> [VTQD_VehActSpd_kph]
  [VTQD_VehActSpd_kph] -> ECO_OnePedal_TqMap/7(VTQD_VehActSpd_kph)
  [VTQD_OPDHoldActRelTq_Nm] -> ECO_OnePedal_TqMap/6(VTQD_OPDHoldActRelTq_Nm)
  [VTQD_OPDHoldEnRel_flg] -> ECO_OnePedal_TqMap/5(VTQD_OPDHoldEnRel_flg)

== system tqd/TQD/TorqueDemand/TorqueModule/DriverWhlTqDem/PedalMapWhlTq/NoLHM/ShiftD/LUT_D_Normal ==
  VTQD_TqTargetShaftSpd_rpm : Inport
  VTQD_ActAPSPosn_pct : Inport  Port=2
  VTQD_RegenMode_enum : Inport  Port=3
  VVMC_EstSlope_Deg : Inport  Port=4
  VTQD_APSReqTimer_s : Inport  Port=5
  VTQD_LowIdleAccPedal_flg : Inport  Port=6
  VTQD_OPDHoldEnRel_flg : Inport  Port=7
  VTQD_OPDHoldActRelTq_Nm : Inport  Port=8
  VTQD_VehActSpd_kph : Inport  Port=9
  Action Port : ActionPort
  Constant : Constant  Value=ENUM_REGENLEVEL_LV1
  Constant1 : Constant  Value=ENUM_REGENLEVEL_LV2
  Constant2 : Constant  Value=ENUM_REGENLEVEL_LV3
  Constant3 : Constant  Value=ENUM_REGENLEVEL_LV4
  Constant4 : Constant  Value=ENUM_REGENLEVEL_LV5
  Constant5 : Constant  Value=ENUM_REGENLEVEL_OPD
  Equal{1..6} (6 alike) : RelationalOperator  Operator===  OutDataTypeStr=boolean  RndMeth=Simplest
  If : If  NumInputs=6  IfExpression=u1 ~= 0  ElseIfExpressions=u2 ~= 0, u3 ~= 0, u4 ~= 0, u5 ~= 0, u6~=0
  MTQD_NL1TqMapD_Z_Nm : Lookup_n-D  BreakpointsForDimension1=ATQD_NL1TqMapD_Y_pct  BreakpointsForDimension2=ATQD_NL1TqMapD_X_rpm  Table=MTQD_NL1TqMapD_Z_Nm  ExtrapMethod=Clip  InternalRulePriority=Speed  RndMeth=Simplest  InputSameDT=on
      settings: InputPortMap=u0,u1
  MTQD_NL2TqMapD_Z_Nm : Lookup_n-D  BreakpointsForDimension1=ATQD_NL1TqMapD_Y_pct  BreakpointsForDimension2=ATQD_NL1TqMapD_X_rpm  Table=MTQD_NL2TqMapD_Z_Nm  ExtrapMethod=Clip  InternalRulePriority=Speed  RndMeth=Simplest  InputSameDT=on
      settings: InputPortMap=u0,u1
  MTQD_NL3TqMapD_Z_Nm : Lookup_n-D  BreakpointsForDimension1=ATQD_NL1TqMapD_Y_pct  BreakpointsForDimension2=ATQD_NL1TqMapD_X_rpm  Table=MTQD_NL3TqMapD_Z_Nm  ExtrapMethod=Clip  InternalRulePriority=Speed  RndMeth=Simplest  InputSameDT=on
      settings: InputPortMap=u0,u1
  MTQD_NL4TqMapD_Z_Nm1 : Lookup_n-D  BreakpointsForDimension1=ATQD_NL1TqMapD_Y_pct  BreakpointsForDimension2=ATQD_NL1TqMapD_X_rpm  Table=MTQD_NL4TqMapD_Z_Nm  ExtrapMethod=Clip  InternalRulePriority=Speed  RndMeth=Simplest  InputSameDT=on
      settings: InputPortMap=u0,u1
  MTQD_NL5TqMapD_Z_Nm1 : Lookup_n-D  BreakpointsForDimension1=ATQD_NL1TqMapD_Y_pct  BreakpointsForDimension2=ATQD_NL1TqMapD_X_rpm  Table=MTQD_NL5TqMapD_Z_Nm  ExtrapMethod=Clip  InternalRulePriority=Speed  RndMeth=Simplest  InputSameDT=on
      settings: InputPortMap=u0,u1
  MTQD_NOPDTqMapDCon_Z_Nm : Lookup_n-D  BreakpointsForDimension1=ATQD_NOPDTqMapDCon_Y_Deg  BreakpointsForDimension2=ATQD_NOPDTqMapDCon_X_rpm  Table=MTQD_NOPDTqMapDCon_Z_Nm  ExtrapMethod=Clip  InternalRulePriority=Speed  RndMeth=Simplest  InputSameDT=on
      settings: InputPortMap=u0,u1
  MTQD_NOPDTqMapD_Z_Nm1 : Lookup_n-D  BreakpointsForDimension1=ATQD_NL1TqMapD_Y_pct  BreakpointsForDimension2=ATQD_NL1TqMapD_X_rpm  Table=MTQD_NOPDTqMapD_Z_Nm  ExtrapMethod=Clip  InternalRulePriority=Speed  RndMeth=Simplest  InputSameDT=on
      settings: InputPortMap=u0,u1
  Merge : Merge  Inputs=7
  NRM_Invalid_TqMap1 : Subsystem  TreatAsAtomicUnit=on
  NRM_Lv1_TqMap : Subsystem  TreatAsAtomicUnit=on
  NRM_Lv2_TqMap : Subsystem  TreatAsAtomicUnit=on
  NRM_Lv3_TqMap : Subsystem  TreatAsAtomicUnit=on
  NRM_Lv4_TqMap : Subsystem  TreatAsAtomicUnit=on
  NRM_Lv5_TqMap : Subsystem  TreatAsAtomicUnit=on
  NRM_OnePedal_TqMap : Subsystem  TreatAsAtomicUnit=on
  VTQD_WhlTqNRMD_Nm : Outport
  wires:
  Equal6/1 -> If/6
  [VTQD_RegenMode_enum] -> Equal6/1
  Constant5/1 -> Equal6/2
  Equal5/1 -> If/5
  [VTQD_RegenMode_enum] -> Equal5/1
  Constant4/1 -> Equal5/2
  Equal4/1 -> If/4
  [VTQD_RegenMode_enum] -> Equal4/1
  Constant3/1 -> Equal4/2
  [VTQD_RegenMode_enum] -> Equal3/1
  Constant2/1 -> Equal3/2
  [VTQD_RegenMode_enum] -> Equal2/1
  Constant1/1 -> Equal2/2
  Constant/1 -> Equal1/2
  [VTQD_RegenMode_enum] -> Equal1/1
  [VTQD_NOPDTqMapD_Nm] -> NRM_OnePedal_TqMap/1(VTQD_NOPDTqMapDIn_Nm)
  If/6 -> NRM_OnePedal_TqMap/Action
  NRM_OnePedal_TqMap/1(VTQD_NOPDTqMapDOut_Nm) -> Merge/6
  [VTQD_NL5TqMapD_Nm] -> NRM_Lv5_TqMap/1(VTQD_NL5TqMapDIn_Nm)
  If/5 -> NRM_Lv5_TqMap/Action
  NRM_Lv5_TqMap/1(VTQD_NL5TqMapDOut_Nm) -> Merge/5
  NRM_Lv4_TqMap/1(VTQD_NL4TqMapDOut_Nm) -> Merge/4
  If/4 -> NRM_Lv4_TqMap/Action
  [VTQD_NL4TqMapD_Nm] -> NRM_Lv4_TqMap/1(VTQD_NL4TqMapDIn_Nm)
  [VTQD_NL3TqMapD_Nm] -> NRM_Lv3_TqMap/1(VTQD_NL3TqMapDIn_Nm)
  If/3 -> NRM_Lv3_TqMap/Action
  NRM_Lv3_TqMap/1(VTQD_NL3TqMapDOut_Nm) -> Merge/3
  [VTQD_NL2TqMapD_Nm] -> NRM_Lv2_TqMap/1(VTQD_NL2TqMapDIn_Nm)
  NRM_Lv2_TqMap/1(VTQD_NL2TqMapDOut_Nm) -> Merge/2
  If/2 -> NRM_Lv2_TqMap/Action
  NRM_Lv1_TqMap/1(VTQD_NL1TqMapDOut_Nm) -> Merge/1
  [VTQD_NL1TqMapD_Nm] -> NRM_Lv1_TqMap/1(VTQD_NL1TqMapDIn_Nm)
  Equal1/1 -> If/1
  Equal2/1 -> If/2
  If/1 -> NRM_Lv1_TqMap/Action
  Merge/1 -> VTQD_WhlTqNRMD_Nm/1
  Equal3/1 -> If/3
  [VTQD_TqTargetShaftSpd_rpm] -> MTQD_NOPDTqMapD_Z_Nm1/2
  [VTQD_ActAPSPosn_pct] -> MTQD_NOPDTqMapD_Z_Nm1/1
  [VTQD_TqTargetShaftSpd_rpm] -> MTQD_NL5TqMapD_Z_Nm1/2
  [VTQD_ActAPSPosn_pct] -> MTQD_NL5TqMapD_Z_Nm1/1
  [VTQD_TqTargetShaftSpd_rpm] -> MTQD_NL3TqMapD_Z_Nm/2
  [VTQD_ActAPSPosn_pct] -> MTQD_NL3TqMapD_Z_Nm/1
  [VTQD_TqTargetShaftSpd_rpm] -> MTQD_NL2TqMapD_Z_Nm/2
  [VTQD_ActAPSPosn_pct] -> MTQD_NL2TqMapD_Z_Nm/1
  MTQD_NL5TqMapD_Z_Nm1/1 -> [VTQD_NL5TqMapD_Nm]
  MTQD_NL4TqMapD_Z_Nm1/1 -> [VTQD_NL4TqMapD_Nm]
  [VTQD_TqTargetShaftSpd_rpm] -> MTQD_NL4TqMapD_Z_Nm1/2
  [VTQD_ActAPSPosn_pct] -> MTQD_NL4TqMapD_Z_Nm1/1
  MTQD_NOPDTqMapD_Z_Nm1/1 -> [VTQD_NOPDTqMapD_Nm]
  MTQD_NL3TqMapD_Z_Nm/1 -> [VTQD_NL3TqMapD_Nm]
  MTQD_NL2TqMapD_Z_Nm/1 -> [VTQD_NL2TqMapD_Nm]
  [VTQD_ActAPSPosn_pct] -> MTQD_NL1TqMapD_Z_Nm/1
  [VTQD_TqTargetShaftSpd_rpm] -> MTQD_NL1TqMapD_Z_Nm/2
  VTQD_RegenMode_enum/1 -> [VTQD_RegenMode_enum]
  VTQD_ActAPSPosn_pct/1 -> [VTQD_ActAPSPosn_pct]
  VTQD_TqTargetShaftSpd_rpm/1 -> [VTQD_TqTargetShaftSpd_rpm]
  MTQD_NL1TqMapD_Z_Nm/1 -> [VTQD_NL1TqMapD_Nm]
  [VTQD_NL1TqMapD_Nm] -> NRM_Invalid_TqMap1/1(VTQD_NL1TqMapDIn_Nm)
  If/7 -> NRM_Invalid_TqMap1/Action
  NRM_Invalid_TqMap1/1(VTQD_NL1TqMapDOut_Nm) -> Merge/7
  [VTQD_TqTargetShaftSpd_rpm] -> MTQD_NOPDTqMapDCon_Z_Nm/2
  [VVMC_EstSlope_Deg] -> MTQD_NOPDTqMapDCon_Z_Nm/1
  MTQD_NOPDTqMapDCon_Z_Nm/1 -> [VTQD_NOPDTqMapDCon_Nm]
  VVMC_EstSlope_Deg/1 -> [VVMC_EstSlope_Deg]
  [VTQD_NOPDTqMapDCon_Nm] -> NRM_OnePedal_TqMap/2(VTQD_NOPDTqMapDCon_Nm)
  [VTQD_APSReqTimer_s] -> NRM_OnePedal_TqMap/3(VTQD_APSReqTimer_s)
  VTQD_APSReqTimer_s/1 -> [VTQD_APSReqTimer_s]
  [VTQD_LowIdleAccPedal_flg] -> NRM_OnePedal_TqMap/4(VTQD_LowIdleAccPedal_flg)
  VTQD_LowIdleAccPedal_flg/1 -> [VTQD_LowIdleAccPedal_flg]
  VTQD_OPDHoldEnRel_flg/1 -> [VTQD_OPDHoldEnRel_flg]
  VTQD_OPDHoldActRelTq_Nm/1 -> [VTQD_OPDHoldActRelTq_Nm]
  VTQD_VehActSpd_kph/1 -> [VTQD_VehActSpd_kph]
  [VTQD_OPDHoldEnRel_flg] -> NRM_OnePedal_TqMap/5(VTQD_OPDHoldEnRel_flg)
  [VTQD_OPDHoldActRelTq_Nm] -> NRM_OnePedal_TqMap/6(VTQD_OPDHoldActRelTq_Nm)
  [VTQD_VehActSpd_kph] -> NRM_OnePedal_TqMap/7(VTQD_VehActSpd_kph)

== system tqd/TQD/TorqueDemand/TorqueModule/DriverWhlTqDem/PedalMapWhlTq/NoLHM/ShiftD/LUT_D_Sport ==
  VTQD_TqTargetShaftSpd_rpm : Inport
  VTQD_ActAPSPosn_pct : Inport  Port=2
  VTQD_RegenMode_enum : Inport  Port=3
  VVMC_EstSlope_Deg : Inport  Port=4
  VTQD_APSReqTimer_s : Inport  Port=5
  VTQD_LowIdleAccPedal_flg : Inport  Port=6
  VTQD_OPDHoldEnRel_flg : Inport  Port=7
  VTQD_OPDHoldActRelTq_Nm : Inport  Port=8
  VTQD_VehActSpd_kph : Inport  Port=9
  Action Port : ActionPort
  Constant : Constant  Value=ENUM_REGENLEVEL_LV1
  Constant1 : Constant  Value=ENUM_REGENLEVEL_LV2
  Constant2 : Constant  Value=ENUM_REGENLEVEL_LV3
  Constant3 : Constant  Value=ENUM_REGENLEVEL_LV4
  Constant4 : Constant  Value=ENUM_REGENLEVEL_LV5
  Constant5 : Constant  Value=ENUM_REGENLEVEL_OPD
  Equal{1..6} (6 alike) : RelationalOperator  Operator===  OutDataTypeStr=boolean  RndMeth=Simplest
  If : If  NumInputs=6  IfExpression=u1 ~= 0  ElseIfExpressions=u2 ~= 0, u3 ~= 0, u4 ~= 0, u5 ~= 0, u6 ~= 0
  MTQD_SL1TqMapD_Z_Nm : Lookup_n-D  BreakpointsForDimension1=ATQD_SL1TqMapD_Y_pct  BreakpointsForDimension2=ATQD_SL1TqMapD_X_rpm  Table=MTQD_SL1TqMapD_Z_Nm  ExtrapMethod=Clip  InternalRulePriority=Speed  RndMeth=Simplest  InputSameDT=on
      settings: InputPortMap=u0,u1
  MTQD_SL2TqMapD_Z_Nm : Lookup_n-D  BreakpointsForDimension1=ATQD_SL1TqMapD_Y_pct  BreakpointsForDimension2=ATQD_SL1TqMapD_X_rpm  Table=MTQD_SL2TqMapD_Z_Nm  ExtrapMethod=Clip  InternalRulePriority=Speed  RndMeth=Simplest  InputSameDT=on
      settings: InputPortMap=u0,u1
  MTQD_SL3TqMapD_Z_Nm : Lookup_n-D  BreakpointsForDimension1=ATQD_SL1TqMapD_Y_pct  BreakpointsForDimension2=ATQD_SL1TqMapD_X_rpm  Table=MTQD_SL3TqMapD_Z_Nm  ExtrapMethod=Clip  InternalRulePriority=Speed  RndMeth=Simplest  InputSameDT=on
      settings: InputPortMap=u0,u1
  MTQD_SL4TqMapD_Z_Nm : Lookup_n-D  BreakpointsForDimension1=ATQD_SL1TqMapD_Y_pct  BreakpointsForDimension2=ATQD_SL1TqMapD_X_rpm  Table=MTQD_SL4TqMapD_Z_Nm  ExtrapMethod=Clip  InternalRulePriority=Speed  RndMeth=Simplest  InputSameDT=on
      settings: InputPortMap=u0,u1
  MTQD_SL5TqMapD_Z_Nm : Lookup_n-D  BreakpointsForDimension1=ATQD_SL1TqMapD_Y_pct  BreakpointsForDimension2=ATQD_SL1TqMapD_X_rpm  Table=MTQD_SL5TqMapD_Z_Nm  ExtrapMethod=Clip  InternalRulePriority=Speed  RndMeth=Simplest  InputSameDT=on
      settings: InputPortMap=u0,u1
  MTQD_SOPDTqMapDCon_Z_Nm : Lookup_n-D  BreakpointsForDimension1=ATQD_SOPDTqMapDCon_Y_Deg  BreakpointsForDimension2=ATQD_SOPDTqMapDCon_X_rpm  Table=MTQD_SOPDTqMapDCon_Z_Nm  ExtrapMethod=Clip  InternalRulePriority=Speed  RndMeth=Simplest  InputSameDT=on
      settings: InputPortMap=u0,u1
  MTQD_SOPDTqMapD_Z_Nm : Lookup_n-D  BreakpointsForDimension1=ATQD_SL1TqMapD_Y_pct  BreakpointsForDimension2=ATQD_SL1TqMapD_X_rpm  Table=MTQD_SOPDTqMapD_Z_Nm  ExtrapMethod=Clip  InternalRulePriority=Speed  RndMeth=Simplest  InputSameDT=on
      settings: InputPortMap=u0,u1
  Merge : Merge  Inputs=7
  Sport_Invalid_TqMap1 : Subsystem  TreatAsAtomicUnit=on
  Sport_Lv1_TqMap : Subsystem  TreatAsAtomicUnit=on
  Sport_Lv2_TqMap : Subsystem  TreatAsAtomicUnit=on
  Sport_Lv3_TqMap : Subsystem  TreatAsAtomicUnit=on
  Sport_Lv4_TqMap : Subsystem  TreatAsAtomicUnit=on
  Sport_Lv5_TqMap : Subsystem  TreatAsAtomicUnit=on
  Sport_OnePedal_TqMap : Subsystem  TreatAsAtomicUnit=on
  VTQD_WhlTqSPORTD_Nm : Outport
  wires:
  Equal6/1 -> If/6
  [VTQD_RegenMode_enum] -> Equal6/1
  Constant5/1 -> Equal6/2
  Equal5/1 -> If/5
  [VTQD_RegenMode_enum] -> Equal5/1
  Constant4/1 -> Equal5/2
  Equal4/1 -> If/4
  [VTQD_RegenMode_enum] -> Equal4/1
  Constant3/1 -> Equal4/2
  [VTQD_RegenMode_enum] -> Equal3/1
  Constant2/1 -> Equal3/2
  [VTQD_RegenMode_enum] -> Equal2/1
  Constant1/1 -> Equal2/2
  Constant/1 -> Equal1/2
  [VTQD_RegenMode_enum] -> Equal1/1
  [VTQD_SOPDTqMapD_Nm] -> Sport_OnePedal_TqMap/1(VTQD_SOPDTqMapDIn_Nm)
  If/6 -> Sport_OnePedal_TqMap/Action
  Sport_OnePedal_TqMap/1(VTQD_SOPDTqMapDOut_Nm) -> Merge/6
  [VTQD_SL5TqMapD_Nm] -> Sport_Lv5_TqMap/1(VTQD_SL5TqMapDIn_Nm)
  If/5 -> Sport_Lv5_TqMap/Action
  Sport_Lv5_TqMap/1(VTQD_SL5TqMapDOut_Nm) -> Merge/5
  Sport_Lv4_TqMap/1(VTQD_SL4TqMapDOut_Nm) -> Merge/4
  If/4 -> Sport_Lv4_TqMap/Action
  [VTQD_SL4TqMapD_Nm] -> Sport_Lv4_TqMap/1(VTQD_SL4TqMapDIn_Nm)
  [VTQD_SL3TqMapD_Nm] -> Sport_Lv3_TqMap/1(VTQD_SL3TqMapDIn_Nm)
  If/3 -> Sport_Lv3_TqMap/Action
  Sport_Lv3_TqMap/1(VTQD_SL3TqMapDOut_Nm) -> Merge/3
  [VTQD_SL2TqMapD_Nm] -> Sport_Lv2_TqMap/1(VTQD_SL2TqMapDIn_Nm)
  Sport_Lv2_TqMap/1(VTQD_SL2TqMapDOut_Nm) -> Merge/2
  If/2 -> Sport_Lv2_TqMap/Action
  Sport_Lv1_TqMap/1(VTQD_SL1TqMapDOut_Nm) -> Merge/1
  [VTQD_SL1TqMapD_Nm] -> Sport_Lv1_TqMap/1(VTQD_SL1TqMapDIn_Nm)
  Equal1/1 -> If/1
  Equal2/1 -> If/2
  If/1 -> Sport_Lv1_TqMap/Action
  Merge/1 -> VTQD_WhlTqSPORTD_Nm/1
  Equal3/1 -> If/3
  [VTQD_TqTargetShaftSpd_rpm] -> MTQD_SOPDTqMapD_Z_Nm/2
  [VTQD_ActAPSPosn_pct] -> MTQD_SOPDTqMapD_Z_Nm/1
  [VTQD_TqTargetShaftSpd_rpm] -> MTQD_SL5TqMapD_Z_Nm/2
  [VTQD_ActAPSPosn_pct] -> MTQD_SL5TqMapD_Z_Nm/1
  [VTQD_TqTargetShaftSpd_rpm] -> MTQD_SL3TqMapD_Z_Nm/2
  [VTQD_ActAPSPosn_pct] -> MTQD_SL3TqMapD_Z_Nm/1
  [VTQD_TqTargetShaftSpd_rpm] -> MTQD_SL2TqMapD_Z_Nm/2
  [VTQD_ActAPSPosn_pct] -> MTQD_SL2TqMapD_Z_Nm/1
  MTQD_SL5TqMapD_Z_Nm/1 -> [VTQD_SL5TqMapD_Nm]
  MTQD_SL4TqMapD_Z_Nm/1 -> [VTQD_SL4TqMapD_Nm]
  [VTQD_TqTargetShaftSpd_rpm] -> MTQD_SL4TqMapD_Z_Nm/2
  [VTQD_ActAPSPosn_pct] -> MTQD_SL4TqMapD_Z_Nm/1
  MTQD_SOPDTqMapD_Z_Nm/1 -> [VTQD_SOPDTqMapD_Nm]
  MTQD_SL3TqMapD_Z_Nm/1 -> [VTQD_SL3TqMapD_Nm]
  MTQD_SL2TqMapD_Z_Nm/1 -> [VTQD_SL2TqMapD_Nm]
  [VTQD_ActAPSPosn_pct] -> MTQD_SL1TqMapD_Z_Nm/1
  [VTQD_TqTargetShaftSpd_rpm] -> MTQD_SL1TqMapD_Z_Nm/2
  VTQD_RegenMode_enum/1 -> [VTQD_RegenMode_enum]
  VTQD_ActAPSPosn_pct/1 -> [VTQD_ActAPSPosn_pct]
  VTQD_TqTargetShaftSpd_rpm/1 -> [VTQD_TqTargetShaftSpd_rpm]
  MTQD_SL1TqMapD_Z_Nm/1 -> [VTQD_SL1TqMapD_Nm]
  [VTQD_SL1TqMapD_Nm] -> Sport_Invalid_TqMap1/1(VTQD_SL1TqMapDIn_Nm)
  If/7 -> Sport_Invalid_TqMap1/Action
  Sport_Invalid_TqMap1/1(VTQD_SL1TqMapDOut_Nm) -> Merge/7
  [VTQD_TqTargetShaftSpd_rpm] -> MTQD_SOPDTqMapDCon_Z_Nm/2
  [VVMC_EstSlope_Deg] -> MTQD_SOPDTqMapDCon_Z_Nm/1
  MTQD_SOPDTqMapDCon_Z_Nm/1 -> [VTQD_SOPDTqMapDCon_Nm]
  VVMC_EstSlope_Deg/1 -> [VVMC_EstSlope_Deg]
  VTQD_APSReqTimer_s/1 -> [VTQD_APSReqTimer_s]
  [VTQD_APSReqTimer_s] -> Sport_OnePedal_TqMap/3(VTQD_APSReqTimer_s)
  [VTQD_SOPDTqMapDCon_Nm] -> Sport_OnePedal_TqMap/2(VTQD_SOPDTqMapDCon_Nm)
  [VTQD_LowIdleAccPedal_flg] -> Sport_OnePedal_TqMap/4(VTQD_LowIdleAccPedal_flg)
  VTQD_LowIdleAccPedal_flg/1 -> [VTQD_LowIdleAccPedal_flg]
  VTQD_OPDHoldEnRel_flg/1 -> [VTQD_OPDHoldEnRel_flg]
  VTQD_VehActSpd_kph/1 -> [VTQD_VehActSpd_kph]
  VTQD_OPDHoldActRelTq_Nm/1 -> [VTQD_OPDHoldActRelTq_Nm]
  [VTQD_OPDHoldEnRel_flg] -> Sport_OnePedal_TqMap/5(VTQD_OPDHoldEnRel_flg)
  [VTQD_OPDHoldActRelTq_Nm] -> Sport_OnePedal_TqMap/6(VTQD_OPDHoldActRelTq_Nm)
  [VTQD_VehActSpd_kph] -> Sport_OnePedal_TqMap/7(VTQD_VehActSpd_kph)

== system tqd/TQD/TorqueDemand/TorqueModule/DriverWhlTqDem/PedalMapWhlTq/NoLHM/ShiftD/LUT_D_ECO/ECO_Invalid_TqMap1 ==
  VTQD_RollRegenEnable_flg : Inport
  MTQD_RollGenMapEL1_Z_Nm : Inport  Port=2
  MTQD_ECOTqMapD_Z_Nm : Inport  Port=3
  Action Port : ActionPort
  Switch : Switch  Criteria=u2 ~= 0
  VTQD_EL1TqMapDOut_Nm : Outport
  wires:
  VTQD_RollRegenEnable_flg/1 -> Switch/2
  MTQD_RollGenMapEL1_Z_Nm/1 -> Switch/1
  MTQD_ECOTqMapD_Z_Nm/1 -> Switch/3
  Switch/1 -> VTQD_EL1TqMapDOut_Nm/1

== system tqd/TQD/TorqueDemand/TorqueModule/DriverWhlTqDem/PedalMapWhlTq/NoLHM/ShiftD/LUT_D_ECO/ECO_Lv1_TqMap ==
  VTQD_RollRegenEnable_flg : Inport
  MTQD_RollGenMapEL1_Z_Nm : Inport  Port=2
  MTQD_ECOTqMapD_Z_Nm : Inport  Port=3
  Action Port : ActionPort
  Switch : Switch  Criteria=u2 ~= 0
  VTQD_EL1TqMapDOut_Nm : Outport
  wires:
  Switch/1 -> VTQD_EL1TqMapDOut_Nm/1
  MTQD_ECOTqMapD_Z_Nm/1 -> Switch/3
  MTQD_RollGenMapEL1_Z_Nm/1 -> Switch/1
  VTQD_RollRegenEnable_flg/1 -> Switch/2

== system tqd/TQD/TorqueDemand/TorqueModule/DriverWhlTqDem/PedalMapWhlTq/NoLHM/ShiftD/LUT_D_ECO/ECO_Lv2_TqMap ==
  VTQD_EL2TqMapDIn_Nm : Inport
  Action Port : ActionPort
  VTQD_EL2TqMapDOut_Nm : Outport
  wires:
  VTQD_EL2TqMapDIn_Nm/1 -> VTQD_EL2TqMapDOut_Nm/1

== system tqd/TQD/TorqueDemand/TorqueModule/DriverWhlTqDem/PedalMapWhlTq/NoLHM/ShiftD/LUT_D_ECO/ECO_Lv3_TqMap ==
  VTQD_EL3TqMapDIn_Nm : Inport
  Action Port : ActionPort
  VTQD_EL3TqMapDOut_Nm : Outport
  wires:
  VTQD_EL3TqMapDIn_Nm/1 -> VTQD_EL3TqMapDOut_Nm/1

== system tqd/TQD/TorqueDemand/TorqueModule/DriverWhlTqDem/PedalMapWhlTq/NoLHM/ShiftD/LUT_D_ECO/ECO_Lv4_TqMap ==
  VTQD_EL4TqMapDIn_Nm : Inport
  Action Port : ActionPort
  VTQD_EL4TqMapDOut_Nm : Outport
  wires:
  VTQD_EL4TqMapDIn_Nm/1 -> VTQD_EL4TqMapDOut_Nm/1

== system tqd/TQD/TorqueDemand/TorqueModule/DriverWhlTqDem/PedalMapWhlTq/NoLHM/ShiftD/LUT_D_ECO/ECO_Lv5_TqMap ==
  VTQD_EL5TqMapDIn_Nm : Inport
  Action Port : ActionPort
  VTQD_EL5TqMapDOut_Nm : Outport
  wires:
  VTQD_EL5TqMapDIn_Nm/1 -> VTQD_EL5TqMapDOut_Nm/1

== system tqd/TQD/TorqueDemand/TorqueModule/DriverWhlTqDem/PedalMapWhlTq/NoLHM/ShiftD/LUT_D_ECO/ECO_OnePedal_TqMap ==
  VTQD_EOPDTqMapDIn_Nm : Inport
  VTQD_EOPDTqMapDCon_Nm : Inport  Port=2
  VTQD_APSReqTimer_s : Inport  Port=3
  VTQD_LowIdleAccPedal_flg : Inport  Port=4
  VTQD_OPDHoldEnRel_flg : Inport  Port=5
  VTQD_OPDHoldActRelTq_Nm : Inport  Port=6
  VTQD_VehActSpd_kph : Inport  Port=7
  Action Port : ActionPort
  AND : Logic  AllPortsSameDT=off  OutDataTypeStr=boolean
  Add : Sum
  Constant1 : Constant  Value=ZERO_FLOAT
  Constant2 : Constant  Value=KTQD_OPDHTqDisComSpd_kph
  Constant3 : Constant  Value=ZERO_FLOAT
  Constant9 : Constant  Value=KTQD_APSReqDelayTime_s
  Detect Increase : simulink/Logic and Bit Operations/Detect Increase  vinit=0.0  OutDataTypeStr=boolean
  Max : MinMax  Function=max  Inputs=2
  OR : Logic  Operator=OR  Inputs=3  AllPortsSameDT=off  OutDataTypeStr=boolean
  Relational Operator : RelationalOperator  Operator=>  OutDataTypeStr=boolean  RndMeth=Simplest
  Relational Operator1 : RelationalOperator  Operator=<  OutDataTypeStr=boolean  RndMeth=Simplest
  Relational Operator2 : RelationalOperator  OutDataTypeStr=boolean  RndMeth=Simplest
  SR_Latch : hcu_lib/Basic_Blocks/SR_Latch
  Switch : Switch  Criteria=u2 > Threshold
  Switch1 : Switch  Criteria=u2 > Threshold
  VTQD_EOPDTqMapDOut_Nm : Outport
  wires:
  Constant1/1 -> Switch/1
  VTQD_EOPDTqMapDCon_Nm/1 -> Switch/3
  VTQD_APSReqTimer_s/1 -> Relational Operator2/1
  Switch/1 -> Add/2
  Constant9/1 -> Relational Operator2/2
  VTQD_EOPDTqMapDIn_Nm/1 -> Add/1
  AND/1 -> Switch/2
  Relational Operator2/1 -> AND/1
  VTQD_LowIdleAccPedal_flg/1 -> [VTQD_LowIdleAccPedal_flg]
  [VTQD_LowIdleAccPedal_flg] -> AND/2
  Constant3/1 -> Relational Operator1/2
  Relational Operator1/1 -> OR/3
  Relational Operator/1 -> OR/2
  VTQD_OPDHoldActRelTq_Nm/1 -> Max/2
  [VTQD_LowIdleAccPedal_flg] -> OR/1
  Max/1 -> Switch1/1
  VTQD_OPDHoldEnRel_flg/1 -> Detect Increase/1
  VTQD_VehActSpd_kph/1 -> Relational Operator/1
  Detect Increase/1 -> SR_Latch/1
  Add/1 -> Relational Operator1/1, Max/1, Switch1/3
  OR/1 -> SR_Latch/2
  SR_Latch/1 -> Switch1/2
  Constant2/1 -> Relational Operator/2
  Switch1/1 -> VTQD_EOPDTqMapDOut_Nm/1

== system tqd/TQD/TorqueDemand/TorqueModule/DriverWhlTqDem/PedalMapWhlTq/NoLHM/ShiftD/LUT_D_Normal/NRM_Invalid_TqMap1 ==
  VTQD_NL1TqMapDIn_Nm : Inport
  Action Port : ActionPort
  VTQD_NL1TqMapDOut_Nm : Outport
  wires:
  VTQD_NL1TqMapDIn_Nm/1 -> VTQD_NL1TqMapDOut_Nm/1

== system tqd/TQD/TorqueDemand/TorqueModule/DriverWhlTqDem/PedalMapWhlTq/NoLHM/ShiftD/LUT_D_Normal/NRM_Lv1_TqMap ==
  VTQD_NL1TqMapDIn_Nm : Inport
  Action Port : ActionPort
  VTQD_NL1TqMapDOut_Nm : Outport
  wires:
  VTQD_NL1TqMapDIn_Nm/1 -> VTQD_NL1TqMapDOut_Nm/1

== system tqd/TQD/TorqueDemand/TorqueModule/DriverWhlTqDem/PedalMapWhlTq/NoLHM/ShiftD/LUT_D_Normal/NRM_Lv2_TqMap ==
  VTQD_NL2TqMapDIn_Nm : Inport
  Action Port : ActionPort
  VTQD_NL2TqMapDOut_Nm : Outport
  wires:
  VTQD_NL2TqMapDIn_Nm/1 -> VTQD_NL2TqMapDOut_Nm/1

== system tqd/TQD/TorqueDemand/TorqueModule/DriverWhlTqDem/PedalMapWhlTq/NoLHM/ShiftD/LUT_D_Normal/NRM_Lv3_TqMap ==
  VTQD_NL3TqMapDIn_Nm : Inport
  Action Port : ActionPort
  VTQD_NL3TqMapDOut_Nm : Outport
  wires:
  VTQD_NL3TqMapDIn_Nm/1 -> VTQD_NL3TqMapDOut_Nm/1

== system tqd/TQD/TorqueDemand/TorqueModule/DriverWhlTqDem/PedalMapWhlTq/NoLHM/ShiftD/LUT_D_Normal/NRM_Lv4_TqMap ==
  VTQD_NL4TqMapDIn_Nm : Inport
  Action Port : ActionPort
  VTQD_NL4TqMapDOut_Nm : Outport
  wires:
  VTQD_NL4TqMapDIn_Nm/1 -> VTQD_NL4TqMapDOut_Nm/1

== system tqd/TQD/TorqueDemand/TorqueModule/DriverWhlTqDem/PedalMapWhlTq/NoLHM/ShiftD/LUT_D_Normal/NRM_Lv5_TqMap ==
  VTQD_NL5TqMapDIn_Nm : Inport
  Action Port : ActionPort
  VTQD_NL5TqMapDOut_Nm : Outport
  wires:
  VTQD_NL5TqMapDIn_Nm/1 -> VTQD_NL5TqMapDOut_Nm/1
